simulink model "Steinwurf2"  (Simulink 7.1)
settings: Solver=ode45  StartTime=0.0  StopTime=4  RelTol=1e-3
libraries: simulink x1
settings Model: Creator=Meisel  LastModifiedBy=Meisel

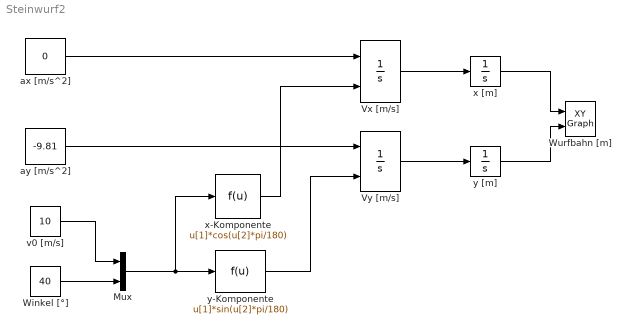
== system Steinwurf2 ==
  Mux : Mux  Inputs=2
  Vx [m/s] : Integrator  InitialConditionSource=external  InitialCondition=5
  Vy [m/s] : Integrator  InitialConditionSource=external  InitialCondition=5
  Winkel [°] : Constant  Value=40  OutDataType=sfix(16)  OutScaling=2^0
  Wurfbahn [m] : simulink/Sinks/XY Graph  SystemSampleTime=-1  xmin=0  xmax=15  ymin=0  ymax=5  st=-1
  ax [m/s^2] : Constant  Value=0  OutDataType=sfix(16)  OutScaling=2^0
  ay [m/s^2] : Constant  Value=-9.81  OutDataType=sfix(16)  OutScaling=2^0
  v0 [m/s] : Constant  Value=10  OutDataType=sfix(16)  OutScaling=2^0
  x [m] : Integrator
  x-Komponente : Fcn  Expr=u[1]*cos(u[2]*pi/180)
  y [m] : Integrator  InitialCondition=1.2
  y-Komponente : Fcn  Expr=u[1]*sin(u[2]*pi/180)
  wires:
  ay [m/s^2]/1 -> Vy [m/s]/1
  Vy [m/s]/1 -> y [m]/1
  ax [m/s^2]/1 -> Vx [m/s]/1
  Vx [m/s]/1 -> x [m]/1
  x [m]/1 -> Wurfbahn [m]/1
  y [m]/1 -> Wurfbahn [m]/2
  Winkel [°]/1 -> Mux/2
  x-Komponente/1 -> Vx [m/s]/2
  y-Komponente/1 -> Vy [m/s]/2
  v0 [m/s]/1 -> Mux/1
  Mux/1 -> x-Komponente/1, y-Komponente/1
